simulink model "SensorModels"  (R2018a)
settings: Solver=VariableStepAuto  StartTime=0.0  StopTime=10.0  RelTol=1e-3
PreLoadFcn:
  | modelDir = fileparts(get_param(bdroot, 'FileName'));
  | addpath(fullfile(modelDir,'../../Parameters'));
  | addpath(fullfile(modelDir,'../../Model/generated'));
  | 
  | Constants_Kugle
  | Parameters_Simulation
InitFcn:
  | Constants_Kugle
  | Parameters_Simulation
undefined symbols (not defined in the file or in its folder): EnableNoise, g, gyro_bias, IMU_height, IMU_misalignment, R_cov_acc, R_cov_gyro, rk, rw, sensor_sigma2_encoder, sensor_sigma2_heading, TicksPrRev, Ts, Ts_heading
libraries: qlib x4, simulink x2
settings Model: Creator=Thomas  LastModifiedBy=Thomas

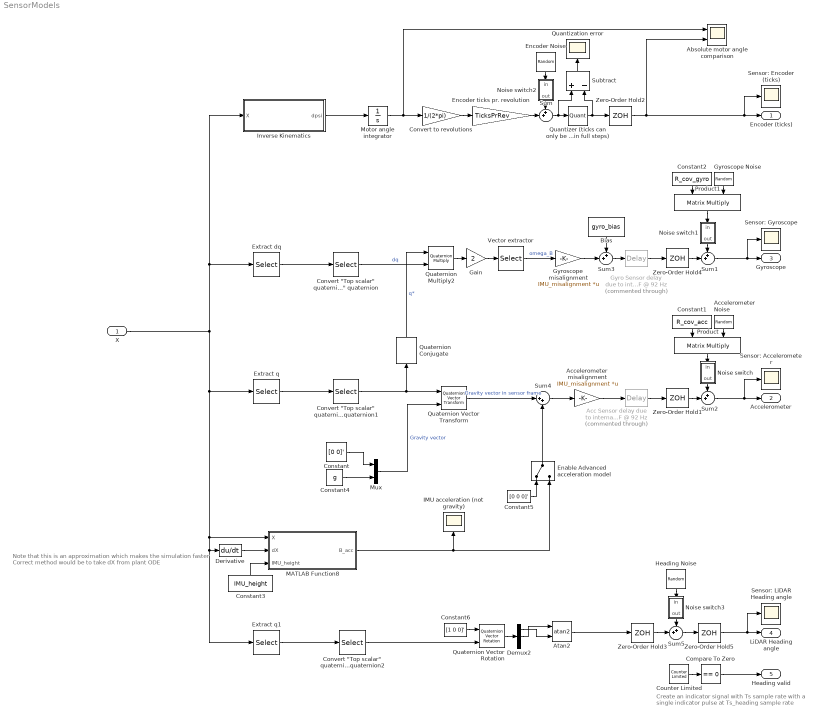
== system SensorModels ==
  note: Create an indicator signal with Ts sample rate with
      | a single indicator pulse at Ts_heading sample rate
  note: Note that this is an approximation which makes the simulation faster
      | Correct method would be to take dX from plant ODE
  X : Inport
  Absolute motor angle comparison : Scope  NumInputPorts=2
  Acc Sensor delay due to internal LPF @ 92 Hz : TransportDelay  Commented=through  DelayTime=7.8e-3  InitialOutput=[0,0,g]'
  Accelerometer Noise : RandomNumber  Mean=[0,0,0]'  Variance=[1,1,1]'  Seed=[31 20 16]'  SampleTime=Ts
  Accelerometer misalignment : Gain  Gain=IMU_misalignment  Multiplication=Matrix(K*u)
  Atan2 : Trigonometry  Operator=atan2
  Bias : Constant  Value=gyro_bias
  Compare To Zero : simulink/Logic and Bit Operations/Compare To Zero  relop===  OutDataTypeStr=boolean
  Constant : Constant  Value=[0 0]'
  Constant1 : Constant  Value=R_cov_acc
  Constant2 : Constant  Value=R_cov_gyro
  Constant3 : Constant  Value=IMU_height
  Constant4 : Constant  Value=g
  Constant5 : Constant  Value=[0 0 0]'
  Constant6 : Constant  Value=[1 0 0]'
  "Convert \"Top scalar\" quaternion to \"Bottom scalar\" quaternion" : Selector  InputPortWidth=4  IndexOptions=Index vector (dialog)  Indices=[2 3 4 1]  OutputSizes=1
  "Convert \"Top scalar\" quaternion to \"Bottom scalar\" quaternion1" : Selector  InputPortWidth=4  IndexOptions=Index vector (dialog)  Indices=[2 3 4 1]  OutputSizes=1
  "Convert \"Top scalar\" quaternion to \"Bottom scalar\" quaternion2" : Selector  InputPortWidth=4  IndexOptions=Index vector (dialog)  Indices=[2 3 4 1]  OutputSizes=1
  Convert to revolutions : Gain  Gain=1/(2*pi)
  Counter Limited : simulink/Sources/Counter Limited  uplimit=Ts_heading/Ts - 1  tsamp=Ts
  Demux2 : Demux  Outputs=3
  Derivative : Derivative
  Enable Advanced acceleration model : ManualSwitch
  Encoder Noise : RandomNumber  Mean=[0,0,0]'  Variance=[sensor_sigma2_encoder, sensor_sigma2_encoder, sensor_sigma2_encoder]'  Seed=[81 9 5]'  SampleTime=Ts
  Encoder ticks pr. revolution : Gain  Gain=TicksPrRev
  Extract dq : Selector  InputPortWidth=12  IndexOptions=Index vector (dialog)  Indices=[9 10 11 12]  OutputSizes=1
  Extract q : Selector  InputPortWidth=12  IndexOptions=Index vector (dialog)  Indices=[3 4 5 6]  OutputSizes=1
  Extract q1 : Selector  InputPortWidth=12  IndexOptions=Index vector (dialog)  Indices=[3 4 5 6]  OutputSizes=1
  Gain : Gain  Gain=2
  Gyro Sensor delay due to internal LPF @ 92 Hz : TransportDelay  Commented=through  DelayTime=3.9e-3
  Gyroscope Noise : RandomNumber  Mean=[0,0,0]'  Variance=[1,1,1]'  Seed=[31 20 16]'  SampleTime=Ts
  Gyroscope misalignment : Gain  Gain=IMU_misalignment  Multiplication=Matrix(K*u)
  Heading Noise : RandomNumber  Variance=sensor_sigma2_heading  Seed=19  SampleTime=Ts_heading
  IMU acceleration (not gravity) : Scope
  Inverse Kinematics : Subsystem
  MATLAB Function8 : MATLAB Function  TreatAsAtomicUnit=on
  Motor angle integrator : Integrator  InitialCondition=[0 0 0]
  Mux : Mux  Inputs=2
  Noise switch : Subsystem
  Noise switch1 : Subsystem
  Noise switch2 : Subsystem
  Noise switch3 : Subsystem
  Product : Product  Multiplication=Matrix(*)
  Product1 : Product  Multiplication=Matrix(*)
  Quantization error : Scope
  Quantizer (ticks can only be measured in full steps) : Quantizer  QuantizationInterval=1
  Quaternion Conjugate : qlib/Quaternion Conjugate
  Quaternion Multiply2 : qlib/Quaternion Multiply
  Quaternion Vector Rotation : qlib/Quaternion Vector Rotation
  Quaternion Vector Transform : qlib/Quaternion Vector Transform
  Sensor: Accelerometer : Scope
  Sensor: Encoder (ticks) : Scope
  Sensor: Gyroscope : Scope
  Sensor: LiDAR Heading angle : Scope
  Subtract : Sum  Inputs=+-
  Sum{,1..3,5} (5 alike) : Sum  Inputs=++|
  Sum4 : Sum  Inputs=|++
  Vector extractor : Selector  InputPortWidth=4  IndexOptions=Index vector (dialog)  Indices=[1 2 3]  OutputSizes=1
  Zero-Order Hold{1..2,4..5} (4 alike) : ZeroOrderHold  SampleTime=Ts
  Zero-Order Hold3 : ZeroOrderHold  SampleTime=Ts_heading
  Encoder (ticks) : Outport
  Accelerometer : Outport  Port=2
  Gyroscope : Outport  Port=3
  LiDAR Heading angle : Outport  Port=4
  Heading valid : Outport  Port=5
  wires:
  Extract q1/1 -> "Convert \"Top scalar\" quaternion to \"Bottom scalar\" quaternion2"/1
  Bias/1 -> Sum3/1
  Accelerometer misalignment/1 -> Acc Sensor delay due to internal LPF @ 92 Hz/1
  Sum5/1 -> Zero-Order Hold5/1
  Quaternion Multiply2/1 -> Gain/1
  Encoder Noise/1 -> Noise switch2/1(in)
  Quaternion Vector Rotation/1 -> Demux2/1
  Atan2/1 -> Zero-Order Hold3/1
  Enable Advanced acceleration model/1 -> Sum4/2
  Demux2/2 -> Atan2/1
  Product/1 -> Noise switch/1(in)
  Vector extractor/1 -> Gyroscope misalignment/1  "omega_B"
  "Convert \"Top scalar\" quaternion to \"Bottom scalar\" quaternion2"/1 -> Quaternion Vector Rotation/2
  Gyroscope misalignment/1 -> Sum3/2
  X/1 -> Inverse Kinematics/1(X), Extract dq/1, MATLAB Function8/1(X), Extract q1/1, Derivative/1, Extract q/1
  Extract dq/1 -> "Convert \"Top scalar\" quaternion to \"Bottom scalar\" quaternion"/1
  Noise switch1/1(out) -> Sum1/1
  Derivative/1 -> MATLAB Function8/2(dX)
  Demux2/1 -> Atan2/2
  Sum/1 -> Subtract/1, Quantizer (ticks can only be measured in full steps)/1
  Product1/1 -> Noise switch1/1(in)
  Encoder ticks pr. revolution/1 -> Sum/2
  Heading Noise/1 -> Noise switch3/1(in)
  Noise switch/1(out) -> Sum2/1
  Sum2/1 -> Sensor: Accelerometer/1, Accelerometer/1
  Quaternion Vector Transform/1 -> Sum4/1  "Gravity vector in sensor frame"
  Constant5/1 -> Enable Advanced acceleration model/1
  MATLAB Function8/1(B_acc) -> Enable Advanced acceleration model/2, IMU acceleration (not gravity)/1
  Subtract/1 -> Quantization error/1
  Sum3/1 -> Gyro Sensor delay due to internal LPF @ 92 Hz/1
  Gyro Sensor delay due to internal LPF @ 92 Hz/1 -> Zero-Order Hold4/1
  Gain/1 -> Vector extractor/1
  Noise switch3/1(out) -> Sum5/1
  Acc Sensor delay due to internal LPF @ 92 Hz/1 -> Zero-Order Hold1/1
  Zero-Order Hold1/1 -> Sum2/2
  Noise switch2/1(out) -> Sum/1
  Constant6/1 -> Quaternion Vector Rotation/1
  Constant3/1 -> MATLAB Function8/3(IMU_height)
  Sum4/1 -> Accelerometer misalignment/1
  Extract q/1 -> "Convert \"Top scalar\" quaternion to \"Bottom scalar\" quaternion1"/1
  Quaternion Conjugate/1 -> Quaternion Multiply2/1  "q*"
  Constant4/1 -> Mux/2
  Convert to revolutions/1 -> Encoder ticks pr. revolution/1
  "Convert \"Top scalar\" quaternion to \"Bottom scalar\" quaternion1"/1 -> Quaternion Vector Transform/1, Quaternion Conjugate/1
  "Convert \"Top scalar\" quaternion to \"Bottom scalar\" quaternion"/1 -> Quaternion Multiply2/2  "dq"
  Motor angle integrator/1 -> Absolute motor angle comparison/1, Convert to revolutions/1
  Zero-Order Hold4/1 -> Sum1/2
  Mux/1 -> Quaternion Vector Transform/2  "Gravity vector"
  Quantizer (ticks can only be measured in full steps)/1 -> Subtract/2, Zero-Order Hold2/1
  Inverse Kinematics/1(dpsi) -> Motor angle integrator/1
  Constant/1 -> Mux/1
  Zero-Order Hold2/1 -> Absolute motor angle comparison/2, Encoder (ticks)/1, Sensor: Encoder (ticks)/1
  Sum1/1 -> Sensor: Gyroscope/1, Gyroscope/1
  Constant1/1 -> Product/1
  Accelerometer Noise/1 -> Product/2
  Gyroscope Noise/1 -> Product1/2
  Constant2/1 -> Product1/1
  Counter Limited/1 -> Compare To Zero/1
  Compare To Zero/1 -> Heading valid/1
  Zero-Order Hold3/1 -> Sum5/2
  Zero-Order Hold5/1 -> Sensor: LiDAR Heading angle/1, LiDAR Heading angle/1

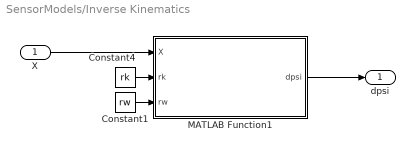
== system SensorModels/Inverse Kinematics ==
  X : Inport
  Constant1 : Constant  Value=rw
  Constant4 : Constant  Value=rk
  MATLAB Function1 : MATLAB Function  TreatAsAtomicUnit=on
  dpsi : Outport
  wires:
  X/1 -> MATLAB Function1/1(X)
  MATLAB Function1/1(dpsi) -> dpsi/1
  Constant1/1 -> MATLAB Function1/3(rw)
  Constant4/1 -> MATLAB Function1/2(rk)

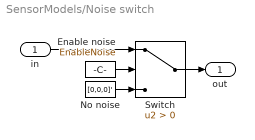
== system SensorModels/Noise switch ==
  in : Inport
  Enable noise : Constant  Value=EnableNoise
  No noise : Constant  Value=[0,0,0]'
  Switch : Switch  Criteria=u2 > Threshold
  out : Outport
  wires:
  No noise/1 -> Switch/3
  Switch/1 -> out/1
  Enable noise/1 -> Switch/2
  in/1 -> Switch/1

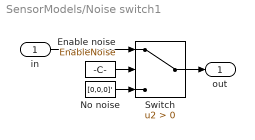
== system SensorModels/Noise switch1 ==
  in : Inport
  Enable noise : Constant  Value=EnableNoise
  No noise : Constant  Value=[0,0,0]'
  Switch : Switch  Criteria=u2 > Threshold
  out : Outport
  wires:
  No noise/1 -> Switch/3
  Switch/1 -> out/1
  Enable noise/1 -> Switch/2
  in/1 -> Switch/1

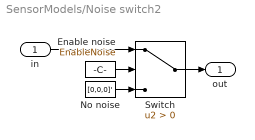
== system SensorModels/Noise switch2 ==
  in : Inport
  Enable noise : Constant  Value=EnableNoise
  No noise : Constant  Value=[0,0,0]'
  Switch : Switch  Criteria=u2 > Threshold
  out : Outport
  wires:
  No noise/1 -> Switch/3
  Switch/1 -> out/1
  Enable noise/1 -> Switch/2
  in/1 -> Switch/1

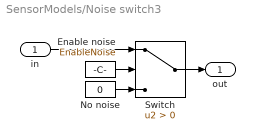
== system SensorModels/Noise switch3 ==
  in : Inport
  Enable noise : Constant  Value=EnableNoise
  No noise : Constant  Value=0
  Switch : Switch  Criteria=u2 > Threshold
  out : Outport
  wires:
  No noise/1 -> Switch/3
  Switch/1 -> out/1
  Enable noise/1 -> Switch/2
  in/1 -> Switch/1

== matlab function SensorModels/Inverse Kinematics/MATLAB Function1 ==
  data: dpsi output; X input; rk input; rw input
function dpsi = InverseKinematics(X,rk,rw)

x = X(1);
y = X(2);
q1 = X(3);
q2 = X(4);
q3 = X(5);
q4 = X(6);

dx = X(7);
dy = X(8);
dq1 = X(9);
dq2 = X(10);
dq3 = X(11);
dq4 = X(12);

dpsi = InverseKinematics(dq1,dq2,dq3,dq4,dx,dy,q1,q2,q3,q4,rk,rw);

== matlab function SensorModels/MATLAB Function8 ==
  data: B_acc output; X input; dX input; IMU_height input
function B_acc = IMU_Acceleration(X,dX,IMU_height)

Phi = @(q)[q(1) -q(2) -q(3) -q(4);     % for q o p = Phi(q) * p
          q(2) q(1)  -q(4) q(3);
          q(3) q(4)  q(1)  -q(2);
          q(4) -q(3) q(2)  q(1)];           
Gamma = @(p)[p(1) -p(2) -p(3) -p(4);   % for q o p = Gamma(p) * q
             p(2) p(1) p(4) -p(3);
             p(3) -p(4) p(1) p(2);
             p(4) p(3) -p(2) p(1)];  

devec = [0,1,0,0;0,0,1,0;0,0,0,1]; % 'v' in notes
vec = [0,0,0;1,0,0;0,1,0;0,0,1]; % '^' in notes

x = X(1);
y = X(2);
q1 = X(3);
q2 = X(4);
q3 = X(5);
q4 = X(6);

dx = X(7);
dy = X(8);
dq1 = X(9);
dq2 = X(10);
dq3 = X(11);
dq4 = X(12);

ddx = dX(7);
ddy = dX(8);
ddq1 = dX(9);
ddq2 = dX(10);
ddq3 = dX(11);
ddq4 = dX(12);

q = X(3:6);
dq = X(9:12);
ddq = dX(9:12);

B_P_IMU = [0;0;IMU_height];
K_P_IMU = devec * Phi(q) * Gamma(q)' * [0;B_P_IMU];
K_dP_IMU = devec * (Phi(dq) * Gamma(q)' + Phi(q) * Gamma(dq)') * [0;B_P_IMU];
K_ddP_IMU = devec * (Phi(ddq) * Gamma(q)' + Phi(dq) * Gamma(dq)') * [0;B_P_IMU]  +  devec * (Phi(dq) * Gamma(dq)' + Phi(q) * Gamma(ddq)') * [0;B_P_IMU];
I_P_IMU = K_P_IMU + [x;y;0];
I_dP_IMU = K_dP_IMU + [dx;dy;0];
I_ddP_IMU = K_ddP_IMU + [ddx;ddy;0];

B_acc = zeros(3,1);
B_acc = devec * Phi(q)' * Gamma(q) * vec * I_ddP_IMU;
